simulink model "local_sequencer_harness"  (R2018b)
settings: Solver=FixedStepDiscrete  StartTime=0  StopTime=11  FixedStep=1  RelTol=1e-3
undefined symbols (not defined in the file or in its folder): eof, sigbuilder_block, sldvsubsys, StateFlowModeType
libraries: sldvlib x21, simulink x6, hdlsllib x4
(part 1 of 2)
settings Model: SldvGeneratedHarnessModel=TestUnitModel=local_sequencer|  Creator=hiterd  LastModifiedBy=gauthamsm
settings DataIOCC: SaveFormat=StructureWithTime
settings OptimizationCC: BlockReduction=off  ConditionallyExecuteInputs=off  DefaultParameterBehavior=Inlined  ExpressionFolding=off
settings DebuggingCC: InheritedTsInSrcMsg=none  LibraryContextMissingDiagnostic=none
settings SFSimCC: SimUseLocalCustomCode=off
settings RTWCC: RTWUseLocalCustomCode=off
settings ConfigComp: DVMode=PropertyProving  DVModelCoverageObjectives=MCDC  DVTestSuiteOptimization=CombinedObjectives (Nonlinear Extended)  DVDetectOutOfBounds=on  DVSaveExpectedOutput=on  DVDisplayReport=off

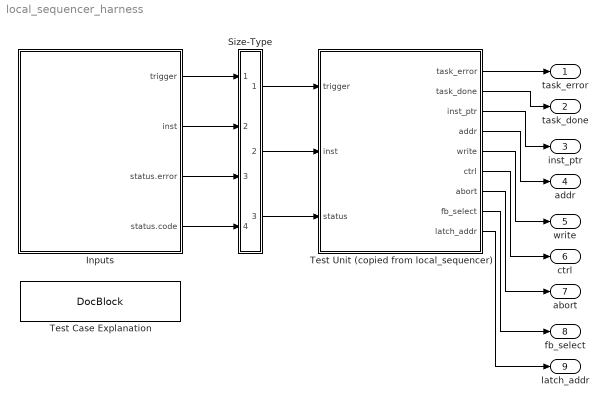
== system local_sequencer_harness ==
  Inputs : Subsystem  Tag=STV Subsys  LoadFcn=sigbuilder_block('load',[50 50 520 400 ]);  StartFcn=sigbuilder_block('start');  StopFcn=sigbuilder_block('stop');  ClipboardFcn=sigbuilder_block('clipboard');  mask(Sigbuilder block){tuvar=[0:10]}
      mask init:
      | if ~strcmp(get_param(bdroot(gcb),'SimulationStatus'),'stopped'),tuvar = sigbuilder_block('maskInit'); end
      settings: CopyFcn=sigbuilder_block('copy');  DeleteFcn=sigbuilder_block('delete');  ModelCloseFcn=sigbuilder_block('modelClose');  PreSaveFcn=sigbuilder_block('preSave');  PauseFcn=sigbuilder_block('pause');  ContinueFcn=sigbuilder_block('continue');  NameChangeFcn=sigbuilder_block('namechange');  OpenFcn=sigbuilder_block('open');  CloseFcn=sigbuilder_block('close');
      mask Display: plot(0, 0, 100, 100,[2, 2, 32, 32, 2], [68, 8, 8, 68, 68],[32, 2], [38, 38], [32, 19, 2],[53, 60, 44], [32, 17, 17, 2],[16, 16, 31, 31]);txt = getActiveGroup(gcbh);text(2, 100, txt,'verticalAlignment', 'top');
  Size-Type : Subsystem
  Test Case Explanation : simulink/Model-Wide Utilities/DocBlock  DocumentType=Text
  Test Unit (copied from local_sequencer) : Subsystem
  task_error : Outport  RequirementInfo={'linktype_rmi_slreq' 'local_sequencer_req.slreqx' '20' 'true' 'ERROR (local_sequencer_req#20)' '' ; 'linktype_rmi_slreq' 'local_sequencer_req.slreqx' '29' 'true' 'Error Signal Service Provided (local_sequencer_req#29)' '' } %GIDa_4b3727b3_eed7_4111_ba54_d506f35d5492  OutDataTypeStr=boolean
  task_done : Outport  RequirementInfo={'linktype_rmi_slreq' 'local_sequencer_req.slreqx' '19' 'true' 'TASK_DONE (local_sequencer_req#19)' '' ; 'linktype_rmi_slreq' 'local_sequencer_req.slreqx' '30' 'true' 'Task Done Service Provided (local_sequencer_req#30)' '' } %GIDa_c01a0f3d_81eb_4c3b_a7a9_b5b96c8ed019  Port=2  OutDataTypeStr=boolean
  inst_ptr : Outport  RequirementInfo={'linktype_rmi_slreq' 'local_sequencer_req.slreqx' '32' 'true' 'Instruction Pointer Service Provided (local_sequencer_req#32)' '' } %GIDa_841fdf6d_6e66_40b6_9879_a3a1e6181a38  Port=3  OutDataTypeStr=task_inst_ptr_type
  addr : Outport  RequirementInfo={'linktype_rmi_slreq' 'local_sequencer_req.slreqx' '31' 'true' 'Task Memory Control Service Provided (local_sequencer_req#31)' '' } %GIDa_8f8748fa_058e_47e8_8fbe_e13b7300a8e2  Port=4  OutMin=[0]  OutDataTypeStr=task_memory_addr_type
  write : Outport  RequirementInfo={'linktype_rmi_slreq' 'local_sequencer_req.slreqx' '17' 'true' 'WRITE (local_sequencer_req#17)' '' ; 'linktype_rmi_slreq' 'local_sequencer_req.slreqx' '31' 'true' 'Task Memory Control Service Provided (local_sequencer_req#31)' '' } %GIDa_4b518ad7_48e7_4af2_afb8_2f880d159183  Port=5  OutDataTypeStr=boolean
  ctrl : Outport  RequirementInfo={'linktype_rmi_slreq' 'local_sequencer_req.slreqx' '15' 'true' 'FETCH (local_sequencer_req#15)' '' ; 'linktype_rmi_slreq' 'local_sequencer_req.slreqx' '16' 'true' 'FB_EXECUTE (local_sequencer_req#16)' '' ; 'linktype_rmi_slreq' 'local_sequencer_req.slreqx' '17' 'true' 'WRITE (local_sequencer_req#17)' '' ; 'linktype_rmi_slreq' 'local_sequencer_req.slreqx' '18' 'true' 'FB_DONE (local_sequencer_req#18)' '' } %GIDa_58b190dd_e50c_4c00_a93b_9cea49031466  Port=6  OutDataTypeStr=boolean
  abort : Outport  RequirementInfo={'linktype_rmi_slreq' 'local_sequencer_req.slreqx' '20' 'true' 'ERROR (local_sequencer_req#20)' '' } %GIDa_8b4e3093_6652_4c1d_818e_447a54a9c3fa  Port=7  OutDataTypeStr=boolean
  fb_select : Outport  RequirementInfo={'linktype_rmi_slreq' 'local_sequencer_req.slreqx' '33' 'true' 'Function Block Selection Service Provided (local_sequencer_req#33)' '' } %GIDa_aec407fa_8f5e_42a9_a8e2_947265fcaaeb  Port=8  OutDataTypeStr=fb_select_type
  latch_addr : Outport  RequirementInfo={} %GIDa_280df430_9f3e_4a55_807b_1e93c9a80428  Port=9  OutMin=[0]  OutDataTypeStr=boolean
  wires:
  Inputs/1(trigger) -> Size-Type/1(In1)
  Size-Type/1(Out1) -> Test Unit (copied from local_sequencer)/1(trigger)
  Inputs/2(inst) -> Size-Type/2(In2)
  Size-Type/2(Out2) -> Test Unit (copied from local_sequencer)/2(inst)
  Inputs/3(status.error) -> Size-Type/3(In5)
  Inputs/4(status.code) -> Size-Type/4(In6)
  Size-Type/3(Out3) -> Test Unit (copied from local_sequencer)/3(status)
  Test Unit (copied from local_sequencer)/1(task_error) -> task_error/1
  Test Unit (copied from local_sequencer)/2(task_done) -> task_done/1
  Test Unit (copied from local_sequencer)/3(inst_ptr) -> inst_ptr/1
  Test Unit (copied from local_sequencer)/4(addr) -> addr/1
  Test Unit (copied from local_sequencer)/5(write) -> write/1
  Test Unit (copied from local_sequencer)/6(ctrl) -> ctrl/1
  Test Unit (copied from local_sequencer)/7(abort) -> abort/1
  Test Unit (copied from local_sequencer)/8(fb_select) -> fb_select/1
  Test Unit (copied from local_sequencer)/9(latch_addr) -> latch_addr/1

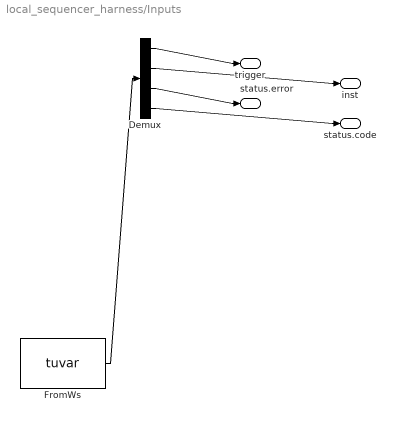
== system local_sequencer_harness/Inputs ==
  Demux : Demux  Tag=STV Demux
  FromWs : FromWorkspace  Tag=STV FromWs  VariableName=tuvar  SampleTime=0
      SigBuilderData=|
      | dataSet(1).timeRange = [0 5]
      | dataSet(1).name = 'Counterexample 1'
      | dataSet(2).timeRange = [0 5]
      | dataSet(2).name = 'Counterexample 2'
      | sbobj.Name = 'Signal Builder'
      | sbobj.Groups(1).Name = 'Counterexample 1'
      | sbobj.Groups(1).Signals(1).Name = 'trigger'
      | sbobj.Groups(1).Signals(1).XData = [0 1 2 3 4 5]
      | sbobj.Groups(1).Signals(1).YData = [1 1 1 1 1 1]
      | sbobj.Groups(1).Signals(2).Name = 'inst'
      | sbobj.Groups(1).Signals(2).XData = [0 1 2 3 4 5]
      | sbobj.Groups(1).Signals(2).YData = [2147483646 2147483646 2147483646 2147483646 2147483646 2147483646]
      | sbobj.Groups(1).Signals(3).Name = 'status.error'
      | sbobj.Groups(1).Signals(3).XData = [0 1 2 3 4 4 5]
      | sbobj.Groups(1).Signals(3).YData = [0 0 0 0 0 1 1]
      | sbobj.Groups(1).Signals(4).Name = 'status.code'
      | sbobj.Groups(1).Signals(4).XData = [0 1 1 2 2 3 3 4 4 5]
      | sbobj.Groups(1).Signals(4).YData = [71303168 71303168 260046849 260046849 524288000 524288000 524288001 524288001 2675965952 2675965952]
      | sbobj.Groups(1).TimeRange = [0 5]
      | sbobj.Groups(2).Name = 'Counterexample 2'
      | sbobj.Groups(2).Signals(1).Name = 'trigger'
      | sbobj.Groups(2).Signals(1).XData = [0 1 2 2 3 3 4 4 5]
      | sbobj.Groups(2).Signals(1).YData = [1 1 1 0 0 1 1 0 0]
      | sbobj.Groups(2).Signals(2).Name = 'inst'
      | sbobj.Groups(2).Signals(2).XData = [0 1 2 3 4 5]
      | sbobj.Groups(2).Signals(2).YData = [2147483646 2147483646 2147483646 2147483646 2147483646 2147483646]
      | sbobj.Groups(2).Signals(3).Name = 'status.error'
      | sbobj.Groups(2).Signals(3).XData = [0 1 2 3 4 4 5]
      | sbobj.Groups(2).Signals(3).YData = [0 0 0 0 0 1 1]
      | sbobj.Groups(2).Signals(4).Name = 'status.code'
      | sbobj.Groups(2).Signals(4).XData = [0 1 1 2 2 3 4 4 5]
      | sbobj.Groups(2).Signals(4).YData = [71303168 71303168 260046848 260046848 524288000 524288000 524288000 2675965953 2675965953]
      | sbobj.Groups(2).TimeRange = [0 5]
  trigger : Outport  Tag=STV Outport
  inst : Outport  Tag=STV Outport  Port=2
  status.error : Outport  Tag=STV Outport  Port=3
  status.code : Outport  Tag=STV Outport  Port=4
  wires:
  FromWs/1 -> Demux/1
  Demux/1 -> trigger/1
  Demux/2 -> inst/1
  Demux/3 -> status.error/1
  Demux/4 -> status.code/1

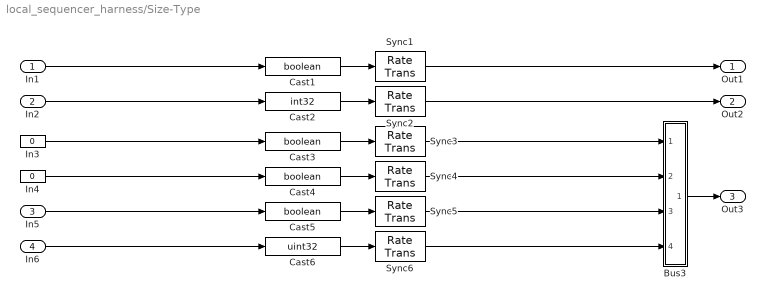
== system local_sequencer_harness/Size-Type ==
  In1 : Inport
  In2 : Inport  Port=2
  In5 : Inport  Port=3
  In6 : Inport  Port=4
  Bus3 : Subsystem
  Cast{1,3..5} (4 alike) : DataTypeConversion  OutDataTypeStr=boolean  RndMeth=Nearest  SaturateOnIntegerOverflow=on
  Cast2 : DataTypeConversion  OutDataTypeStr=int32  RndMeth=Nearest  SaturateOnIntegerOverflow=on
  Cast6 : DataTypeConversion  OutDataTypeStr=uint32  RndMeth=Nearest  SaturateOnIntegerOverflow=on
  In3 : Constant  Value=0  OutDataTypeStr=double
  In4 : Constant  Value=0  OutDataTypeStr=double
  Sync{1..6} (6 alike) : RateTransition  OutPortSampleTime=[1,0]
  Out1 : Outport
  Out2 : Outport  Port=2
  Out3 : Outport  Port=3
  wires:
  In1/1 -> Cast1/1
  Cast1/1 -> Sync1/1
  Sync1/1 -> Out1/1
  In2/1 -> Cast2/1
  Cast2/1 -> Sync2/1
  Sync2/1 -> Out2/1
  In3/1 -> Cast3/1
  Cast3/1 -> Sync3/1
  In4/1 -> Cast4/1
  Cast4/1 -> Sync4/1
  In5/1 -> Cast5/1
  Cast5/1 -> Sync5/1
  In6/1 -> Cast6/1
  Cast6/1 -> Sync6/1
  Sync3/1 -> Bus3/1(status(1).done)
  Sync4/1 -> Bus3/2(status(1).busy)
  Sync5/1 -> Bus3/3(status(1).error)
  Sync6/1 -> Bus3/4(status(1).code)
  Bus3/1(Out) -> Out3/1

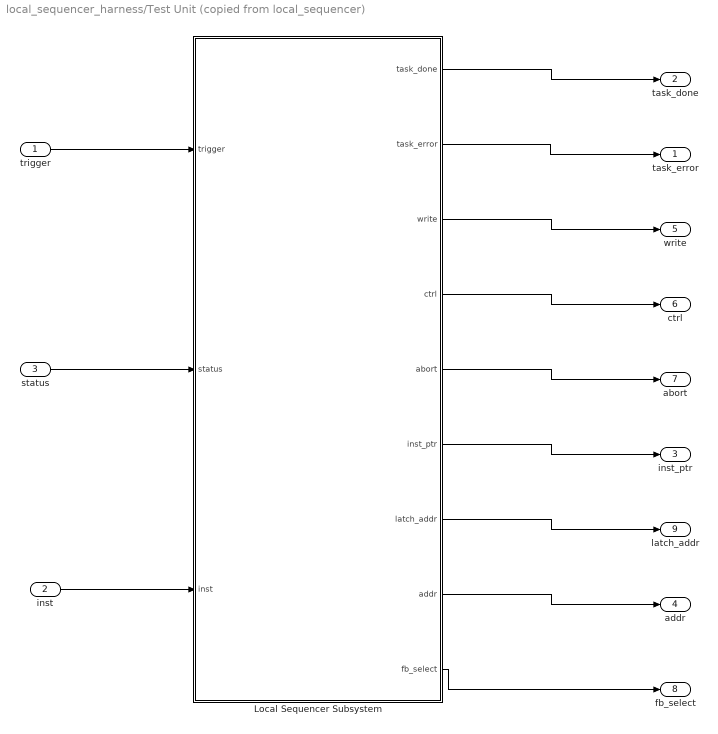
== system local_sequencer_harness/Test Unit (copied from local_sequencer) ==
  trigger : Inport  RequirementInfo={'linktype_rmi_slreq' 'local_sequencer_req.slreqx' '1' 'true' 'Trigger Service Received (local_sequencer_req#1)' '' } %GIDa_4d9765d8_c1f7_44d1_847e_63d15330923d  OutDataTypeStr=boolean  SampleTime=1
  inst : Inport  RequirementInfo={'linktype_rmi_slreq' 'local_sequencer_req.slreqx' '2' 'true' 'Instruction Service Received (local_sequencer_req#2)' '' } %GIDa_6e08ed8d_7128_4ad3_9be2_20afc87b0780  Port=2  OutDataTypeStr=task_inst_data_type  SampleTime=1
  status : Inport  RequirementInfo={'linktype_rmi_slreq' 'local_sequencer_req.slreqx' '3' 'true' 'Function Block Status Service Received (local_sequencer_req#3)' '' } %GIDa_a844bf10_1c01_4e71_b367_abd6e060c4a4  Port=3  OutDataTypeStr=Bus: fb_status  SampleTime=1
  Local Sequencer Subsystem : Subsystem  RequirementInfo={} %GIDa_691ea0b4_f849_451b_b844_cf268bee6922
  task_error : Outport  RequirementInfo={'linktype_rmi_slreq' 'local_sequencer_req.slreqx' '20' 'true' 'ERROR (local_sequencer_req#20)' '' ; 'linktype_rmi_slreq' 'local_sequencer_req.slreqx' '29' 'true' 'Error Signal Service Provided (local_sequencer_req#29)' '' } %GIDa_e9ce8bc7_3977_4377_8523_e6d870486e24  OutDataTypeStr=boolean
  task_done : Outport  RequirementInfo={'linktype_rmi_slreq' 'local_sequencer_req.slreqx' '19' 'true' 'TASK_DONE (local_sequencer_req#19)' '' ; 'linktype_rmi_slreq' 'local_sequencer_req.slreqx' '30' 'true' 'Task Done Service Provided (local_sequencer_req#30)' '' } %GIDa_4f63a98d_be6f_4c69_865c_747d34c7a994  Port=2  OutDataTypeStr=boolean
  inst_ptr : Outport  RequirementInfo={'linktype_rmi_slreq' 'local_sequencer_req.slreqx' '32' 'true' 'Instruction Pointer Service Provided (local_sequencer_req#32)' '' } %GIDa_ae4a976f_0dc8_4a2d_b976_c9d40035a665  Port=3  OutDataTypeStr=task_inst_ptr_type
  addr : Outport  RequirementInfo={'linktype_rmi_slreq' 'local_sequencer_req.slreqx' '31' 'true' 'Task Memory Control Service Provided (local_sequencer_req#31)' '' } %GIDa_c8e29bee_29f9_4d2c_a739_7a936b29a70c  Port=4  OutMin=[0]  OutDataTypeStr=task_memory_addr_type
  write : Outport  RequirementInfo={'linktype_rmi_slreq' 'local_sequencer_req.slreqx' '17' 'true' 'WRITE (local_sequencer_req#17)' '' ; 'linktype_rmi_slreq' 'local_sequencer_req.slreqx' '31' 'true' 'Task Memory Control Service Provided (local_sequencer_req#31)' '' } %GIDa_a08e580f_e59d_4d36_808e_415d3b412f66  Port=5  OutDataTypeStr=boolean
  ctrl : Outport  RequirementInfo={'linktype_rmi_slreq' 'local_sequencer_req.slreqx' '15' 'true' 'FETCH (local_sequencer_req#15)' '' ; 'linktype_rmi_slreq' 'local_sequencer_req.slreqx' '16' 'true' 'FB_EXECUTE (local_sequencer_req#16)' '' ; 'linktype_rmi_slreq' 'local_sequencer_req.slreqx' '17' 'true' 'WRITE (local_sequencer_req#17)' '' ; 'linktype_rmi_slreq' 'local_sequencer_req.slreqx' '18' 'true' 'FB_DONE (local_sequencer_req#18)' '' } %GIDa_798b687a_16a8_42b6_9002_483e38f3c64e  Port=6  OutDataTypeStr=boolean
  abort : Outport  RequirementInfo={'linktype_rmi_slreq' 'local_sequencer_req.slreqx' '20' 'true' 'ERROR (local_sequencer_req#20)' '' } %GIDa_0f3d61c3_2d7b_4dce_ac88_a1459569f952  Port=7  OutDataTypeStr=boolean
  fb_select : Outport  RequirementInfo={'linktype_rmi_slreq' 'local_sequencer_req.slreqx' '33' 'true' 'Function Block Selection Service Provided (local_sequencer_req#33)' '' } %GIDa_2bafbd9a_e614_424c_a6eb_704ceba625c2  Port=8  OutDataTypeStr=fb_select_type
  latch_addr : Outport  RequirementInfo={} %GIDa_f6d0df7c_bed9_4f3c_a302_54711bc6950e  Port=9  OutMin=[0]  OutDataTypeStr=boolean
  wires:
  trigger/1 -> Local Sequencer Subsystem/1(trigger)
  status/1 -> Local Sequencer Subsystem/2(status)
  inst/1 -> Local Sequencer Subsystem/3(inst)
  Local Sequencer Subsystem/1(task_done) -> task_done/1
  Local Sequencer Subsystem/2(task_error) -> task_error/1
  Local Sequencer Subsystem/3(write) -> write/1
  Local Sequencer Subsystem/4(ctrl) -> ctrl/1
  Local Sequencer Subsystem/5(abort) -> abort/1
  Local Sequencer Subsystem/6(inst_ptr) -> inst_ptr/1
  Local Sequencer Subsystem/7(latch_addr) -> latch_addr/1
  Local Sequencer Subsystem/8(addr) -> addr/1
  Local Sequencer Subsystem/9(fb_select) -> fb_select/1

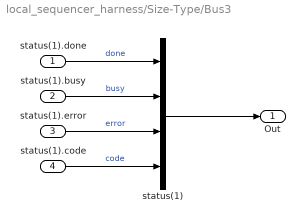
== system local_sequencer_harness/Size-Type/Bus3 ==
  status(1).done : Inport
  status(1).busy : Inport  Port=2
  status(1).error : Inport  Port=3
  status(1).code : Inport  Port=4
  status(1) : BusCreator  Inputs=4  OutDataTypeStr=Bus: fb_status
  Out : Outport
  wires:
  status(1).done/1 -> status(1)/1  "done"
  status(1).busy/1 -> status(1)/2  "busy"
  status(1).error/1 -> status(1)/3  "error"
  status(1).code/1 -> status(1)/4  "code"
  status(1)/1 -> Out/1

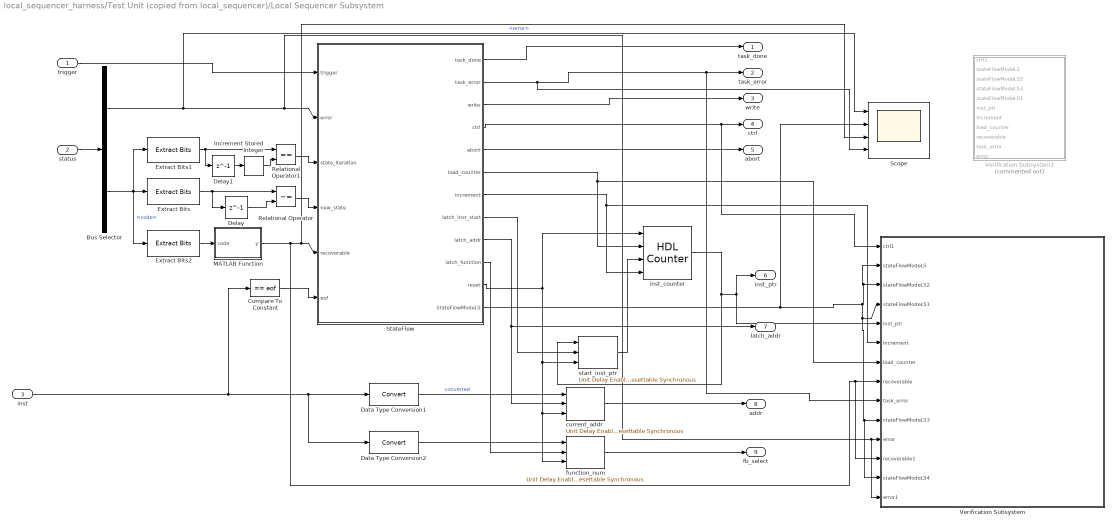
== system local_sequencer_harness/Test Unit (copied from local_sequencer)/Local Sequencer Subsystem ==
  trigger : Inport  RequirementInfo={} %GIDa_1e8ca34a_c9d3_45ae_b0e7_559df57917bf
  status : Inport  RequirementInfo={} %GIDa_1a7e6c0b_3888_45e7_9699_00d25f52f0df  Port=2
  inst : Inport  RequirementInfo={} %GIDa_cf2bd6e1_6b2b_450c_945a_cc71645fdc78  Port=3
  Bus Selector : BusSelector  RequirementInfo={} %GIDa_a162605f_6826_4012_8456_0f670d372e3e  OutputSignals=error,code
  Compare To Constant : simulink/Logic and Bit Operations/Compare To Constant  RequirementInfo={'linktype_rmi_slreq' 'local_sequencer_req.slreqx' '7' 'true' 'End of File Determination (local_sequencer_req#7)' '' } %GIDa_1bfea16f_c62a_4475_9710_996025bad8c0  relop===  const=eof  OutDataTypeStr=boolean
  Data Type Conversion1 : DataTypeConversion  RequirementInfo={'linktype_rmi_slreq' 'local_sequencer_req.slreqx' '34' 'true' 'Conversion of Data Input (local_sequencer_req#34)' '' } %GIDa_bcea22fb_1305_4e6d_9be5_7c5894791e9c
  Data Type Conversion2 : DataTypeConversion  RequirementInfo={'linktype_rmi_slreq' 'local_sequencer_req.slreqx' '34' 'true' 'Conversion of Data Input (local_sequencer_req#34)' '' } %GIDa_b03bb29e_727f_4560_91c2_987e1544289f
  Delay : Delay  RequirementInfo={'linktype_rmi_slreq' 'local_sequencer_req.slreqx' '5' 'true' 'Super State Change Detection (local_sequencer_req#5)' '' } %GIDa_826e27ed_e26c_448f_bb39_3b3ecfac7830  DelayLength=1
  Delay1 : Delay  RequirementInfo={'linktype_rmi_slreq' 'local_sequencer_req.slreqx' '4' 'true' 'Super State Iteration Detection (local_sequencer_req#4)' '' } %GIDa_9af56f70_0ad9_4e15_b1d3_d222492c0231  DelayLength=1
  Extract Bits : simulink/Logic and Bit Operations/Extract Bits  RequirementInfo={'linktype_rmi_slreq' 'local_sequencer_req.slreqx' '5' 'true' 'Super State Change Detection (local_sequencer_req#5)' '' } %GIDa_ed216d48_4236_4a6e_94ae_32688075c1c1  bitsToExtract=Range starting with most significant bit  numBits=4  bitIdxRange=[0 7]  outScalingMode=Treat bit field as an integer
      settings: SourceProductName=Simulink
  Extract Bits1 : simulink/Logic and Bit Operations/Extract Bits  RequirementInfo={'linktype_rmi_slreq' 'local_sequencer_req.slreqx' '4' 'true' 'Super State Iteration Detection (local_sequencer_req#4)' '' } %GIDa_f8a72584_cc2f_4dda_9538_a363ad475483  bitsToExtract=Range of bits  numBits=4  bitIdxRange=[22 27]  outScalingMode=Treat bit field as an integer
      settings: SourceProductName=Simulink
  Extract Bits2 : simulink/Logic and Bit Operations/Extract Bits  RequirementInfo={'linktype_rmi_slreq' 'local_sequencer_req.slreqx' '6' 'true' 'Error Recovery Determination (local_sequencer_req#6)' '' } %GIDa_6508cd16_8925_49b2_89d0_f2044608e5fd  bitsToExtract=Range ending with least significant bit  numBits=22  bitIdxRange=[22 27]  outScalingMode=Treat bit field as an integer
      settings: SourceProductName=Simulink
  Increment Stored Integer : simulink/Additional Math & Discrete/Additional Math: Increment - Decrement/Increment Stored Integer  RequirementInfo={'linktype_rmi_slreq' 'local_sequencer_req.slreqx' '4' 'true' 'Super State Iteration Detection (local_sequencer_req#4)' '' } %GIDa_eff492e6_55b4_4f8f_bf38_25fea0c3ba44
      settings: SourceProductName=Simulink
  MATLAB Function : MATLAB Function  RequirementInfo={'linktype_rmi_slreq' 'local_sequencer_req.slreqx' '6' 'true' 'Error Recovery Determination (local_sequencer_req#6)' '' } %GIDa_0e0ae0c6_7f44_44d8_8ce2_7f424de04522  TreatAsAtomicUnit=on
  Relational Operator : RelationalOperator  RequirementInfo={'linktype_rmi_slreq' 'local_sequencer_req.slreqx' '5' 'true' 'Super State Change Detection (local_sequencer_req#5)' '' } %GIDa_c7a5acef_9ee6_48bf_acb3_5cd08911dcb3  Operator=~=  OutDataTypeStr=boolean  RndMeth=Nearest
  Relational Operator1 : RelationalOperator  RequirementInfo={'linktype_rmi_slreq' 'local_sequencer_req.slreqx' '4' 'true' 'Super State Iteration Detection (local_sequencer_req#4)' '' } %GIDa_e00291a7_d6c4_4999_8243_fd86dde3d581  Operator===  OutDataTypeStr=boolean  RndMeth=Nearest
  Scope : Scope  NumInputPorts=4
      settings: RequirementInfo={} %GIDa_a27e6c01_8b88_4284_ab1b_80a338979146
  StateFlow : Stateflow chart  RequirementInfo={'linktype_rmi_slreq' 'local_sequencer_req.slreqx' '12' 'true' 'Controller Super States (local_sequencer_req#12)' '' } %GIDa_cc643d51_32d6_41cb_beee_853cbc937ec5  TreatAsAtomicUnit=on
  Verification Subsystem : Subsystem  Tag=VerificationSubsystem  RequirementInfo={} %GIDa_b9231509_133e_4ec9_afa8_12fadf576824  DisableCoverage=on  LoadFcn=sldvsubsys('check')  TreatAsAtomicUnit=on  SimViewingDevice=on  mask(VerificationSubsystem){}
      mask init:
      | sldvsubsys('maskInit');
      settings: CopyFcn=sldvsubsys('copy');  OpenFcn=open_system(gcb,'force');
      settings: PreSaveFcn=|
      | set_param(gcb,'SimViewingDevice','on');
      | sldvsubsys('check');
      mask Help: helpview(fullfile(docroot,'toolbox','sldv','sldv.map'),'verificationsubsystem')
      mask Display: image(imread('sldvicon_versubsys.png','BackGroundColor',[1 1 1]),'center');
  Verification Subsystem1 : Subsystem  Tag=VerificationSubsystem  RequirementInfo={} %GIDa_b5211482_203e_477a_a04f_44f6097f9954  Commented=on  DisableCoverage=on  LoadFcn=sldvsubsys('check')  TreatAsAtomicUnit=on  SimViewingDevice=on  mask(VerificationSubsystem){}
      mask init:
      | sldvsubsys('maskInit');
      settings: CopyFcn=sldvsubsys('copy');  OpenFcn=open_system(gcb,'force');
      settings: PreSaveFcn=|
      | set_param(gcb,'SimViewingDevice','on');
      | sldvsubsys('check');
      mask Help: helpview(fullfile(docroot,'toolbox','sldv','sldv.map'),'verificationsubsystem')
      mask Display: image(imread('sldvicon_versubsys.png','BackGroundColor',[1 1 1]),'center');
  current_addr : hdlsllib/Discrete/Unit Delay Enabled Resettable Synchronous  RequirementInfo={'linktype_rmi_slreq' 'local_sequencer_req.slreqx' '11' 'true' 'Current Address Register (local_sequencer_req#11)' '' } %GIDa_b8f7f4f3_37ca_4546_8bdc_9675d816c663  InitialCondition=0  SampleTime=-1
      settings: SourceProductName=HDL Coder  SourceProductBaseCode=HD
  function_num : hdlsllib/Discrete/Unit Delay Enabled Resettable Synchronous  RequirementInfo={'linktype_rmi_slreq' 'local_sequencer_req.slreqx' '8' 'true' 'Function Number Register (local_sequencer_req#8)' '' } %GIDa_658e3425_55a5_4c8c_8b70_ff26cff3d567  InitialCondition=0  SampleTime=-1
      settings: SourceProductName=HDL Coder  SourceProductBaseCode=HD
  inst_counter : hdlsllib/Sources/HDL Counter  RequirementInfo={'linktype_rmi_slreq' 'local_sequencer_req.slreqx' '10' 'true' 'Instruction Counter (local_sequencer_req#10)' '' } %GIDa_4f8fbdf8_b7e8_445f_8c6c_70eaab5f3fef  CountType=Free running  CountInit=0  CountStep=1  CountMax=25  CountFromType=Initial value  CountFrom=0  CountResetPort=on  CountLoadPort=on  CountEnbPort=on  CountDirPort=off  CountDataType=Unsigned  CountWordLen=32  CountFracLen=0  CountSampTime=1
      settings: SourceProductBaseCode=HD
  start_inst_ptr : hdlsllib/Discrete/Unit Delay Enabled Resettable Synchronous  RequirementInfo={'linktype_rmi_slreq' 'local_sequencer_req.slreqx' '9' 'true' 'Start Instruction Pointer Register (local_sequencer_req#9)' '' } %GIDa_059fbd8a_63b8_486f_a2ee_beef95e9e77a  InitialCondition=0  SampleTime=-1
      settings: SourceProductName=HDL Coder  SourceProductBaseCode=HD
  task_done : Outport  RequirementInfo={} %GIDa_742b0145_7b38_4077_85b0_9b3c6bbcc75a
  task_error : Outport  RequirementInfo={} %GIDa_20ca7631_3271_4d84_8143_ec18b5855ad9  Port=2
  write : Outport  RequirementInfo={} %GIDa_15c2c95f_69ed_4817_8697_d9e8efe15443  Port=3
  ctrl : Outport  RequirementInfo={} %GIDa_ab925feb_6031_4560_b0bf_8fccdac808d1  Port=4
  abort : Outport  RequirementInfo={} %GIDa_af91d9c3_b667_48b7_844a_d06301abb7fe  Port=5
  inst_ptr : Outport  RequirementInfo={} %GIDa_92246ee0_b390_431d_84f7_855d2625f298  Port=6
  latch_addr : Outport  RequirementInfo={} %GIDa_c018af9e_064e_4093_9f4e_4119ccab6bc1  Port=7
  addr : Outport  RequirementInfo={} %GIDa_55309190_ab2c_44a1_af5f_111a38240509  Port=8
  fb_select : Outport  RequirementInfo={} %GIDa_d0ad82d1_5299_4359_b05c_642c3938d8a5  Port=9
  wires:
  StateFlow/12(StateFlowModeLS) -> Verification Subsystem/2(stateFlowModeLS), Verification Subsystem/3(stateFlowModeLS2), Verification Subsystem/4(stateFlowModeLS1), Verification Subsystem/10(stateFlowModeLS3), Verification Subsystem/13(stateFlowModeLS4), Scope/2
  StateFlow/3(write) -> write/1
  current_addr/1 -> addr/1
  StateFlow/4(ctrl) -> ctrl/1, Verification Subsystem/1(ctrl1)
  StateFlow/1(task_done) -> task_done/1
  trigger/1 -> StateFlow/1(trigger)
  Extract Bits/1 -> Delay/1, Relational Operator/1
  MATLAB Function/1(y) -> StateFlow/5(recoverable), Scope/3, Verification Subsystem/8(recoverable), Verification Subsystem/12(recoverable1)
  StateFlow/10(latch_function) -> function_num/2
  Data Type Conversion2/1 -> function_num/1
  Relational Operator1/1 -> StateFlow/3(state_iteration)
  Delay/1 -> Relational Operator/2
  StateFlow/2(task_error) -> task_error/1, Verification Subsystem/9(task_error), Scope/4
  function_num/1 -> fb_select/1
  inst/1 -> Compare To Constant/1, Data Type Conversion2/1, Data Type Conversion1/1
  Compare To Constant/1 -> StateFlow/6(eof)
  Relational Operator/1 -> StateFlow/4(new_state)
  Bus Selector/1 -> StateFlow/2(error), Verification Subsystem/11(error), Verification Subsystem/14(error1), Scope/1  "<error>"
  inst_counter/1 -> start_inst_ptr/1, inst_ptr/1, Verification Subsystem/5(inst_ptr)
  Increment Stored Integer/1 -> Relational Operator1/2
  Delay1/1 -> Increment Stored Integer/1
  StateFlow/5(abort) -> abort/1
  Extract Bits1/1 -> Relational Operator1/1, Delay1/1
  Extract Bits2/1 -> MATLAB Function/1(code)
  Bus Selector/2 -> Extract Bits/1, Extract Bits1/1, Extract Bits2/1  "<code>"
  StateFlow/6(load_counter) -> inst_counter/2, Verification Subsystem/7(load_counter)
  StateFlow/11(reset) -> inst_counter/1, start_inst_ptr/3, current_addr/3, function_num/3
  start_inst_ptr/1 -> inst_counter/3
  Data Type Conversion1/1 -> current_addr/1  "converted"
  status/1 -> Bus Selector/1
  StateFlow/7(increment) -> inst_counter/4, Verification Subsystem/6(increment)
  StateFlow/8(latch_inst_start) -> start_inst_ptr/2
  StateFlow/9(latch_addr) -> current_addr/2, latch_addr/1

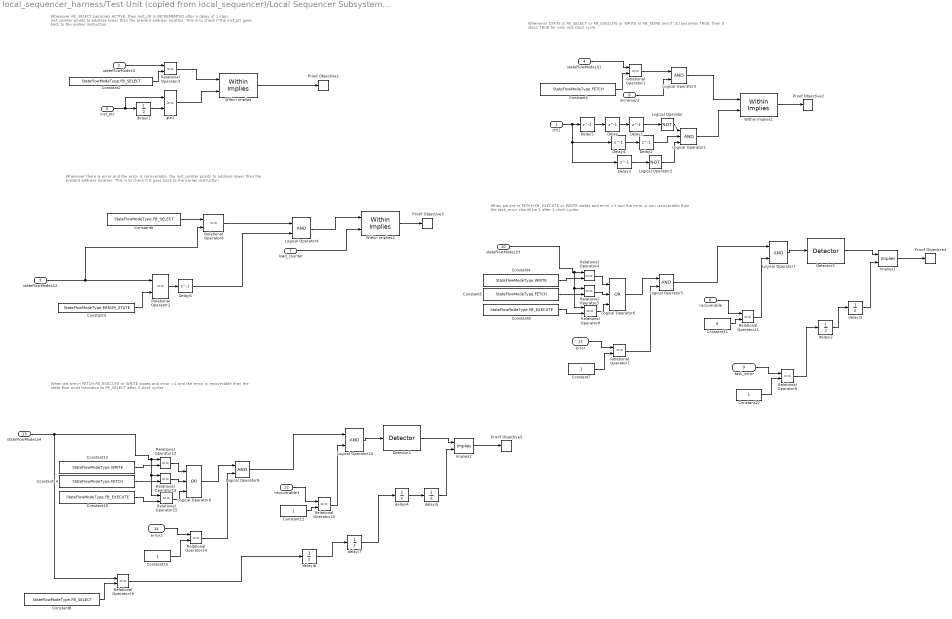
== system local_sequencer_harness/Test Unit (copied from local_sequencer)/Local Sequencer Subsystem/Verification Subsystem ==
  note: When we are in FETCH,FB_EXECUTE or WRITE states and error =1 and the error is
      | recoverable then the state flow must transition to FB_SELECT after 3 clock cycles
  note: When we are in FETCH,FB_EXECUTE or WRITE states and error =1 and the error is non
      | recoverable then the task_error should be 1 after 2 clock cycles
  note: Whenever there is error and the error is recoverable, the inst_pointer points to address lower than the present address location. This is to check if it goes back to the earlier instruction
  note: Whenever STATE is FB_SELECT or FB_EXECUTE or WRITE or FB_DONE and if ctrl becomes TRUE, then it stays TRUE for only one clock cycle.
  note: Whenever FB_SELECT becomes ACTIVE, then inst_ptr is INCREMENTED after a delay of 1 step. inst_pointer points to address lower than the present address location. This is to check if the inst_ptr goes back to the earlier instruction
  ctrl1 : Inport  RequirementInfo={} %GIDa_6b645b52_a750_41af_9a8f_c377cd2cb97e
  stateFlowModeLS : Inport  RequirementInfo={} %GIDa_a4712168_761f_42ae_85b8_8ff9b981d0c1  Port=2  OutDataTypeStr=Enum: StateFlowModeType
  stateFlowModeLS2 : Inport  RequirementInfo={} %GIDa_a7c47b6a_432f_4217_84f3_98ed5b16bf25  Port=3  OutDataTypeStr=Enum: StateFlowModeType
  stateFlowModeLS1 : Inport  RequirementInfo={} %GIDa_5f3d4289_f256_4d9b_bbfa_4cb2e9ba7701  Port=4  OutDataTypeStr=Enum: StateFlowModeType
  inst_ptr : Inport  RequirementInfo={} %GIDa_c73084db_e622_4a82_be5c_67d8c46f613f  Port=5
  increment : Inport  RequirementInfo={} %GIDa_34715739_1965_4b88_a576_10e1b9c7bcf1  Port=6
  load_counter : Inport  RequirementInfo={} %GIDa_5349dcb2_c6d2_4b2e_b931_b803d0eafd2b  Port=7
  recoverable : Inport  RequirementInfo={} %GIDa_52514d1c_d4b4_450c_86d9_102baf416947  Port=8
  task_error : Inport  RequirementInfo={} %GIDa_964329ab_c3cb_483d_bd3e_3f8fce772734  Port=9
  stateFlowModeLS3 : Inport  RequirementInfo={} %GIDa_9f2c847c_a6f0_4dc8_bb70_fd807a5031c3  Port=10  OutDataTypeStr=Enum: StateFlowModeType
  error : Inport  RequirementInfo={} %GIDa_04b1a319_44c2_495c_839e_7cc0812e627f  Port=11
  recoverable1 : Inport  RequirementInfo={} %GIDa_8b8bdee0_7233_4c53_b78f_8a52cb74d75c  Port=12
  stateFlowModeLS4 : Inport  RequirementInfo={} %GIDa_8e458654_ea3c_4d4d_a88e_c6df996ebab2  Port=13  OutDataTypeStr=Enum: StateFlowModeType
  error1 : Inport  RequirementInfo={} %GIDa_44510cdf_839a_486d_8342_15fd6b9a6cb1  Port=14
  Constant1 : Constant  RequirementInfo={} %GIDa_6342d419_8342_43a0_919e_6a27c2e3eafb  Value=StateFlowModeType.FETCH
  Constant10 : Constant  RequirementInfo={} %GIDa_71987e0a_f819_4bc1_ae0f_86cb959ba58c
  Constant11 : Constant  RequirementInfo={} %GIDa_53afce07_30fd_4890_a83f_b84bd58684b9  Value=0
  Constant12 : Constant  RequirementInfo={} %GIDa_03f01666_acfc_4a3b_baa9_c0a59d7d126e
  Constant13 : Constant  RequirementInfo={} %GIDa_e2c573b3_bc29_4365_a3fd_1284c1938177  Value=StateFlowModeType.WRITE
  Constant14 : Constant  RequirementInfo={} %GIDa_779f599a_1458_40c4_9c18_37dc7796f943  Value=StateFlowModeType.FETCH
  Constant15 : Constant  RequirementInfo={} %GIDa_dcb54f72_e8f5_4e18_8b8c_1ce10482da3a
  Constant16 : Constant  RequirementInfo={} %GIDa_e11c02e6_61a8_4c9a_98bf_78bf0f833513  Value=StateFlowModeType.FB_EXECUTE
  Constant2 : Constant  RequirementInfo={} %GIDa_d77b991c_77a2_43c8_ba8b_1d5970f428ac  Value=StateFlowModeType.FB_SELECT
  Constant3 : Constant  RequirementInfo={} %GIDa_d4a9d497_af6c_46f0_916a_43b417355251  Value=StateFlowModeType.ERROR_STATE
  Constant4 : Constant  RequirementInfo={} %GIDa_1e8e59d8_61df_4eca_8fc5_fa09a17b912f  Value=StateFlowModeType.WRITE
  Constant5 : Constant  RequirementInfo={} %GIDa_aae79a7f_f71c_4685_826d_81802dfd129c  Value=StateFlowModeType.FETCH
  Constant6 : Constant  RequirementInfo={} %GIDa_0c059a54_d970_4c46_8833_35b3baf3127a  Value=StateFlowModeType.FB_SELECT
  Constant7 : Constant  RequirementInfo={} %GIDa_a0429521_ac1f_4e13_ac01_d69038e9b625
  Constant8 : Constant  RequirementInfo={} %GIDa_ccd36f88_2729_4a8b_ae6c_3d5c45613874  Value=StateFlowModeType.FB_SELECT
  Constant9 : Constant  RequirementInfo={} %GIDa_e96794ef_4892_4db9_b2c5_07e7e6a3d411  Value=StateFlowModeType.FB_EXECUTE
  Delay : Delay  RequirementInfo={} %GIDa_81740ed4_2784_46f4_85c1_6dbb980f36f6  DelayLength=1  InitialCondition=0
  Delay1 : Delay  RequirementInfo={} %GIDa_dffa4db5_9115_4a6c_bc24_8c31b2b0ae2a  DelayLength=1  InitialCondition=0
  Delay2 : Delay  RequirementInfo={} %GIDa_2b4b34b7_28e3_4da6_9c5c_4161cd76c929  DelayLength=1  InitialCondition=0
  Delay3 : Delay  RequirementInfo={} %GIDa_270c8dcf_c5d6_488c_ab8a_01f21eeed551  DelayLength=1  InitialCondition=0
  Delay4 : Delay  RequirementInfo={} %GIDa_dbf84748_c074_4f31_a9ee_19102cc2667d  DelayLength=1  InitialCondition=0
  Delay5 : Delay  RequirementInfo={} %GIDa_a0fa6fc2_72eb_4e0f_a7af_2b7f78e5a878  DelayLength=1  InitialCondition=0
  Delay6 : Delay  RequirementInfo={} %GIDa_5fa518e1_4830_403b_ae9c_a2474cbcca20  DelayLength=1  InitialCondition=0
  Detector1 : sldvlib/Temporal Operators/Detector  RequirementInfo={} %GIDa_c502c215_ee6c_43d8_964a_396c216b10d4  reset=off  typ=Synchronized  in_hold=1  delay=0  out_hold=5
      settings: SourceProductName=Simulink Design Verifier  SourceProductBaseCode=DV
  Detector3 : sldvlib/Temporal Operators/Detector  RequirementInfo={} %GIDa_429b4896_adea_437f_bd01_5c74a7223186  reset=off  typ=Synchronized  in_hold=1  delay=0  out_hold=5
      settings: SourceProductName=Simulink Design Verifier  SourceProductBaseCode=DV
  Implies1 : sldvlib/Verification Utilities/Implies  RequirementInfo={} %GIDa_bcc7acba_1732_4f58_86db_9c51ed75f38e
      settings: SourceProductName=Simulink Design Verifier  SourceProductBaseCode=DV
  Implies2 : sldvlib/Verification Utilities/Implies  RequirementInfo={} %GIDa_3da248e8_263d_4261_900c_bf2069b027ae
      settings: SourceProductName=Simulink Design Verifier  SourceProductBaseCode=DV
  Logical Operator : Logic  RequirementInfo={} %GIDa_c6ed2fd7_7032_49f1_a73b_59b232d92cfa  Operator=NOT  AllPortsSameDT=off  OutDataTypeStr=boolean
  Logical Operator1 : Logic  RequirementInfo={} %GIDa_11b62c84_4c5b_4fff_b035_221ee7236042  Inputs=3  AllPortsSameDT=off  OutDataTypeStr=boolean
  Logical Operator10 : Logic  RequirementInfo={} %GIDa_82e77056_138f_472c_b35d_04f729bcb552  AllPortsSameDT=off  OutDataTypeStr=boolean
  Logical Operator2 : Logic  RequirementInfo={} %GIDa_bee70a3f_34a4_42dd_b4fe_8c7d25cafb6e  Operator=NOT  AllPortsSameDT=off  OutDataTypeStr=boolean
  Logical Operator3 : Logic  RequirementInfo={} %GIDa_c04f8a76_e51d_4572_9eaa_1319f3d004e1  AllPortsSameDT=off  OutDataTypeStr=boolean
  Logical Operator4 : Logic  RequirementInfo={} %GIDa_ab3c7ee4_4ec3_48d2_9d3e_592908a914fb  AllPortsSameDT=off  OutDataTypeStr=boolean
  Logical Operator5 : Logic  RequirementInfo={} %GIDa_ca91440f_2aa8_4db9_ae7e_a8e1b3d85a5f  AllPortsSameDT=off  OutDataTypeStr=boolean
  Logical Operator6 : Logic  RequirementInfo={} %GIDa_4e9b8a00_7f15_48ae_9c5a_83dd16d3023f  Operator=OR  Inputs=3  AllPortsSameDT=off  OutDataTypeStr=boolean
  Logical Operator7 : Logic  RequirementInfo={} %GIDa_d4822b1c_c277_4986_8ef2_0ba86d669a9a  AllPortsSameDT=off  OutDataTypeStr=boolean
  Logical Operator8 : Logic  RequirementInfo={} %GIDa_59985dd0_0c9a_462a_968b_9254ac594ae7  AllPortsSameDT=off  OutDataTypeStr=boolean
  Logical Operator9 : Logic  RequirementInfo={} %GIDa_0dbbede8_9d83_420c_8489_53d8464b74de  Operator=OR  Inputs=3  AllPortsSameDT=off  OutDataTypeStr=boolean
  Proof Objective1 : sldvlib/Objectives and Constraints/Proof Objective  RequirementInfo={} %GIDa_5a0a3da4_26cd_474e_a9c3_b72501387497  enabled=on  customAVTBlockType=Proof Objective  intervals=true  dispValues=on  outEnabled=off  enableStopSim=off
      settings: AttributesFormatString=%<intervals>  SourceProductName=Simulink Design Verifier  SourceProductBaseCode=DV
  Proof Objective2 : sldvlib/Objectives and Constraints/Proof Objective  RequirementInfo={} %GIDa_d2226da2_0640_43ab_b532_66cb5d7be1b4  enabled=on  customAVTBlockType=Proof Objective  intervals=true  dispValues=on  outEnabled=off  enableStopSim=off
      settings: AttributesFormatString=%<intervals>  SourceProductName=Simulink Design Verifier  SourceProductBaseCode=DV
  Proof Objective3 : sldvlib/Objectives and Constraints/Proof Objective  RequirementInfo={} %GIDa_01fe3c8b_43be_4698_aaaa_97b4f297ef17  enabled=on  customAVTBlockType=Proof Objective  intervals=true  dispValues=on  outEnabled=off  enableStopSim=off
      settings: AttributesFormatString=%<intervals>  SourceProductName=Simulink Design Verifier  SourceProductBaseCode=DV
  Proof Objective4 : sldvlib/Objectives and Constraints/Proof Objective  RequirementInfo={} %GIDa_9469e876_a232_4cd3_b85f_012dd7833a7e  enabled=on  customAVTBlockType=Proof Objective  intervals=true  dispValues=on  outEnabled=off  enableStopSim=off
      settings: AttributesFormatString=%<intervals>  SourceProductName=Simulink Design Verifier  SourceProductBaseCode=DV
  Proof Objective5 : sldvlib/Objectives and Constraints/Proof Objective  RequirementInfo={} %GIDa_7d698c32_5674_4f5c_b6ac_03b8d8626e4d  enabled=on  customAVTBlockType=Proof Objective  intervals=true  dispValues=on  outEnabled=off  enableStopSim=off
      settings: AttributesFormatString=%<intervals>  SourceProductName=Simulink Design Verifier  SourceProductBaseCode=DV
  Relational Operator1 : RelationalOperator  RequirementInfo={} %GIDa_05c76a94_f4f3_4cb4_bfc3_a5737cdb0e00  Operator===  OutDataTypeStr=boolean  RndMeth=Nearest
  Relational Operator10 : RelationalOperator  RequirementInfo={} %GIDa_b5a4404b_9d12_499e_828e_45d226915324  Operator===  OutDataTypeStr=boolean  RndMeth=Nearest
  Relational Operator11 : RelationalOperator  RequirementInfo={} %GIDa_79c55e8f_6948_466a_9872_f547b9db4009  Operator===  OutDataTypeStr=boolean  RndMeth=Nearest
  Relational Operator12 : RelationalOperator  RequirementInfo={} %GIDa_17dec814_d961_4d3d_8cbf_fa9266c87c06  Operator===  OutDataTypeStr=boolean  RndMeth=Nearest
  Relational Operator13 : RelationalOperator  RequirementInfo={} %GIDa_77fa023d_9866_4d25_9e46_7da0f793e291  Operator===  OutDataTypeStr=boolean  RndMeth=Nearest
  Relational Operator14 : RelationalOperator  RequirementInfo={} %GIDa_d8f24c82_795e_4b5f_afa4_92e1340ebe13  Operator===  OutDataTypeStr=boolean  RndMeth=Nearest
  Relational Operator15 : RelationalOperator  RequirementInfo={} %GIDa_2e585a3d_30e2_4ac9_a524_28fc8b3f154b  Operator===  OutDataTypeStr=boolean  RndMeth=Nearest
  Relational Operator16 : RelationalOperator  RequirementInfo={} %GIDa_169954ed_64e0_40c9_accf_05b4d0a779dc  Operator===  OutDataTypeStr=boolean  RndMeth=Nearest
  Relational Operator2 : RelationalOperator  RequirementInfo={} %GIDa_74ed7b7b_e9e7_4b22_946c_9a0b388b4fd8  Operator===  OutDataTypeStr=boolean  RndMeth=Nearest
  Relational Operator3 : RelationalOperator  RequirementInfo={} %GIDa_d53e0909_38f3_4a1d_8d9d_2e2631c0bfd2  Operator===  OutDataTypeStr=boolean  RndMeth=Nearest
  Relational Operator4 : RelationalOperator  RequirementInfo={} %GIDa_b8bcb513_88af_4013_889f_2f7ba0e9afaa  Operator===  OutDataTypeStr=boolean  RndMeth=Nearest
  Relational Operator5 : RelationalOperator  RequirementInfo={} %GIDa_eae57311_6411_4570_9c95_6b21eeb45d86  Operator===  OutDataTypeStr=boolean  RndMeth=Nearest
  Relational Operator6 : RelationalOperator  RequirementInfo={} %GIDa_1a62504d_ac96_482e_ab94_0f36d2b37e2d  Operator===  OutDataTypeStr=boolean  RndMeth=Nearest
  Relational Operator7 : RelationalOperator  RequirementInfo={} %GIDa_c4efe30a_0353_437b_9881_24a86806ccce  Operator===  OutDataTypeStr=boolean  RndMeth=Nearest
  Relational Operator8 : RelationalOperator  RequirementInfo={} %GIDa_cbaf56e6_f0e0_4f5e_b0b1_1a89243fe511  Operator===  OutDataTypeStr=boolean  RndMeth=Nearest
  Relational Operator9 : RelationalOperator  RequirementInfo={} %GIDa_c7d52145_ac3e_4695_87e6_c47e08f80099  Operator===  OutDataTypeStr=boolean  RndMeth=Nearest
  Within Implies : sldvlib/Temporal Operators/Within Implies  RequirementInfo={} %GIDa_a850aec6_0f3a_409f_8ce3_0a4a0710d585  reset=off
      settings: SourceProductName=Simulink Design Verifier  SourceProductBaseCode=DV
  Within Implies1 : sldvlib/Temporal Operators/Within Implies  RequirementInfo={} %GIDa_a8c917f6_d6d4_49b6_a1ef_704c4073a93d  reset=off
      settings: SourceProductName=Simulink Design Verifier  SourceProductBaseCode=DV
  Within Implies2 : sldvlib/Temporal Operators/Within Implies  RequirementInfo={} %GIDa_5f44b74a_97d1_42a0_89ae_0fe79d0dd3f7  reset=off
      settings: SourceProductName=Simulink Design Verifier  SourceProductBaseCode=DV
  delayi1 : UnitDelay  RequirementInfo={} %GIDa_80ccc962_1e13_4ea5_8d86_e8a3cb862295  SampleTime=-1
  delayi2 : UnitDelay  RequirementInfo={} %GIDa_3b80eefc_c665_43bd_a5e3_3099e9de69d6  SampleTime=-1
  delayi3 : UnitDelay  RequirementInfo={} %GIDa_55d82d50_db91_437f_9a22_205827f00855  SampleTime=-1
  delayi4 : UnitDelay  RequirementInfo={} %GIDa_44646075_a9d3_4536_a4bb_2518e6127793  SampleTime=-1
  delayi5 : UnitDelay  RequirementInfo={} %GIDa_0913cb33_ff78_4736_9780_cf397ecef2d2  SampleTime=-1
  delayi6 : UnitDelay  RequirementInfo={} %GIDa_3e1d6896_ec7e_43d0_b858_377f9cbac27f  SampleTime=-1
  delayi7 : UnitDelay  RequirementInfo={} %GIDa_0eb5f02a_08dc_4a81_9a61_1e5499803556  SampleTime=-1
  gte1 : RelationalOperator  RequirementInfo={} %GIDa_58fdfaba_dbdd_4d96_820b_985e384d75dc  OutDataTypeStr=boolean  RndMeth=Nearest
  wires:
  delayi7/1 -> delayi4/1
  delayi6/1 -> delayi7/1
  Relational Operator16/1 -> delayi6/1
  delayi2/1 -> delayi3/1
  Relational Operator9/1 -> delayi2/1
  Constant12/1 -> Relational Operator10/2
  Relational Operator13/1 -> Logical Operator9/2
  Logical Operator8/1 -> Logical Operator10/1
  recoverable1/1 -> Relational Operator10/1
  Relational Operator14/1 -> Logical Operator8/2
  error1/1 -> Relational Operator14/1
  Implies2/1 -> Proof Objective5/1
  delayi5/1 -> Implies2/2
  Relational Operator12/1 -> Logical Operator9/1
  Detector1/1 -> Implies2/1
  Constant13/1 -> Relational Operator12/2
  Constant16/1 -> Relational Operator15/2
  Constant14/1 -> Relational Operator13/2
  Constant15/1 -> Relational Operator14/2
  Logical Operator9/1 -> Logical Operator8/1
  Logical Operator10/1 -> Detector1/1
  Relational Operator15/1 -> Logical Operator9/3
  Constant8/1 -> Relational Operator16/2
  delayi4/1 -> delayi5/1
  stateFlowModeLS4/1 -> Relational Operator16/1, Relational Operator12/1, Relational Operator13/1, Relational Operator15/1
  Relational Operator10/1 -> Logical Operator10/2
  Constant10/1 -> Relational Operator9/2
  task_error/1 -> Relational Operator9/1
  delayi3/1 -> Implies1/2
  Relational Operator11/1 -> Logical Operator7/2
  Logical Operator5/1 -> Logical Operator7/1
  Relational Operator7/1 -> Logical Operator5/2
  Constant7/1 -> Relational Operator7/2
  error/1 -> Relational Operator7/1
  Logical Operator6/1 -> Logical Operator5/1
  Relational Operator8/1 -> Logical Operator6/3
  Relational Operator5/1 -> Logical Operator6/2
  Relational Operator4/1 -> Logical Operator6/1
  Constant9/1 -> Relational Operator8/2
  Constant5/1 -> Relational Operator5/2
  Constant4/1 -> Relational Operator4/2
  stateFlowModeLS3/1 -> Relational Operator4/1, Relational Operator5/1, Relational Operator8/1
  Within Implies1/1 -> Proof Objective2/1
  Within Implies2/1 -> Proof Objective3/1
  Within Implies/1 -> Proof Objective1/1
  Detector3/1 -> Implies1/1
  Logical Operator7/1 -> Detector3/1
  recoverable/1 -> Relational Operator11/1
  Constant11/1 -> Relational Operator11/2
  Implies1/1 -> Proof Objective4/1
  load_counter/1 -> Within Implies2/2
  Constant6/1 -> Relational Operator6/1
  stateFlowModeLS2/1 -> Relational Operator2/1, Relational Operator6/2
  Constant3/1 -> Relational Operator2/2
  Relational Operator2/1 -> Delay6/1
  Relational Operator6/1 -> Logical Operator4/1
  Delay6/1 -> Logical Operator4/2
  Logical Operator4/1 -> Within Implies2/1
  Delay3/1 -> Logical Operator2/1
  Logical Operator3/1 -> Within Implies1/1
  Logical Operator1/1 -> Within Implies1/2
  Delay/1 -> Delay1/1
  Delay4/1 -> Delay2/1
  Relational Operator1/1 -> Logical Operator3/1
  Logical Operator2/1 -> Logical Operator1/3
  Delay2/1 -> Logical Operator1/2
  Constant1/1 -> Relational Operator1/2
  Delay5/1 -> Delay/1
  ctrl1/1 -> Delay5/1, Delay3/1, Delay4/1
  Delay1/1 -> Logical Operator/1
  stateFlowModeLS1/1 -> Relational Operator1/1
  increment/1 -> Logical Operator3/2
  Logical Operator/1 -> Logical Operator1/1
  inst_ptr/1 -> gte1/1, delayi1/1
  stateFlowModeLS/1 -> Relational Operator3/1
  delayi1/1 -> gte1/2
  Constant2/1 -> Relational Operator3/2
  gte1/1 -> Within Implies/2
  Relational Operator3/1 -> Within Implies/1

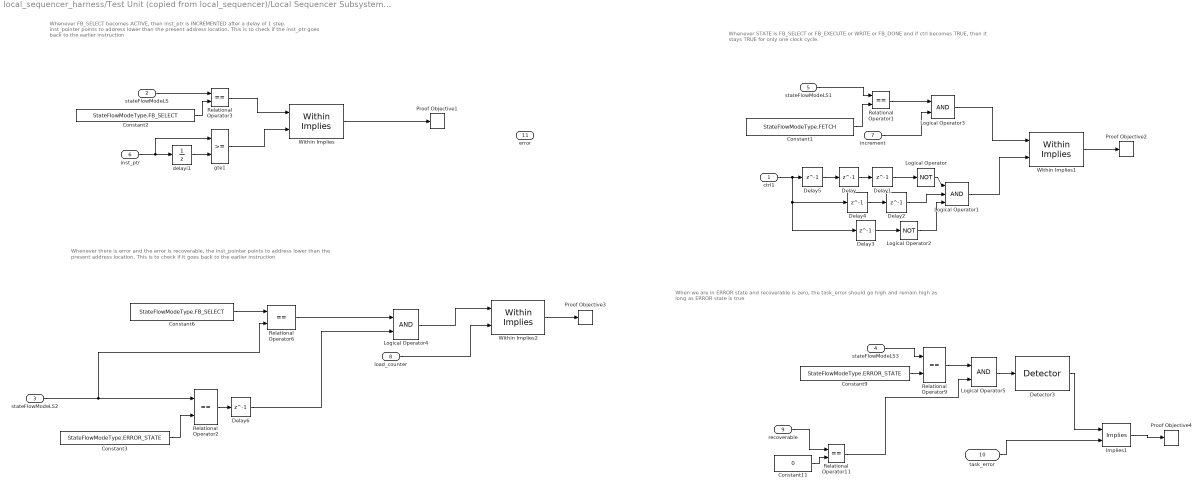
== system local_sequencer_harness/Test Unit (copied from local_sequencer)/Local Sequencer Subsystem/Verification Subsystem1 ==
  note: When we are in ERROR state and recoverable is zero, the task_error should go high and remain high as
      | long as ERROR state is true
  note: Whenever there is error and the error is recoverable, the inst_pointer points to address lower than the present address location. This is to check if it goes back to the earlier instruction
  note: Whenever STATE is FB_SELECT or FB_EXECUTE or WRITE or FB_DONE and if ctrl becomes TRUE, then it stays TRUE for only one clock cycle.
  note: Whenever FB_SELECT becomes ACTIVE, then inst_ptr is INCREMENTED after a delay of 1 step. inst_pointer points to address lower than the present address location. This is to check if the inst_ptr goes back to the earlier instruction
  ctrl1 : Inport  RequirementInfo={} %GIDa_da28b243_b868_43d7_ba2e_8c485d30471d
  stateFlowModeLS : Inport  RequirementInfo={} %GIDa_b658f277_eb35_4939_8a1c_f7bdb11b2e37  Port=2  OutDataTypeStr=Enum: StateFlowModeType
  stateFlowModeLS2 : Inport  RequirementInfo={} %GIDa_9494c7c7_948a_4f36_b45e_b32d219d933d  Port=3  OutDataTypeStr=Enum: StateFlowModeType
  stateFlowModeLS3 : Inport  RequirementInfo={} %GIDa_51971e87_c921_4f6d_98bc_24a46f192aa0  Port=4  OutDataTypeStr=Enum: StateFlowModeType
  stateFlowModeLS1 : Inport  RequirementInfo={} %GIDa_2205d377_0539_4f39_aa27_513b353afdfa  Port=5  OutDataTypeStr=Enum: StateFlowModeType
  inst_ptr : Inport  RequirementInfo={} %GIDa_e0198642_4de5_496c_8a1b_c80b9607f051  Port=6
  increment : Inport  RequirementInfo={} %GIDa_12f780a5_e4a5_4935_a5af_104c2ffef915  Port=7
  load_counter : Inport  RequirementInfo={} %GIDa_20c74391_262e_46b5_99fc_00060d204b47  Port=8
  recoverable : Inport  RequirementInfo={} %GIDa_767ccaa8_8cf2_4dec_8143_5926768f8cf1  Port=9
  task_error : Inport  RequirementInfo={} %GIDa_53cc32c6_315f_4191_931e_4b42866cfb7f  Port=10
  error : Inport  RequirementInfo={} %GIDa_d743bdee_6228_48aa_9015_424286047a7c  Port=11
  Constant1 : Constant  RequirementInfo={} %GIDa_08c62f4c_79dd_4aa1_8e1d_b7672b522beb  Value=StateFlowModeType.FETCH
  Constant11 : Constant  RequirementInfo={} %GIDa_e923a475_eeaa_4f5f_9d1f_bc779aa5a92f  Value=0
  Constant2 : Constant  RequirementInfo={} %GIDa_bdd20e68_8245_43a2_aee1_92fa65b992f0  Value=StateFlowModeType.FB_SELECT
  Constant3 : Constant  RequirementInfo={} %GIDa_32f9eb2f_8c35_4daf_a56f_79bbd1b75113  Value=StateFlowModeType.ERROR_STATE
  Constant6 : Constant  RequirementInfo={} %GIDa_22319c0a_c7bd_46dc_8f0e_1c43c9fbcbe1  Value=StateFlowModeType.FB_SELECT
  Constant9 : Constant  RequirementInfo={} %GIDa_a586b303_ff66_423a_928b_95e4785a77dc  Value=StateFlowModeType.ERROR_STATE
  Delay : Delay  RequirementInfo={} %GIDa_52c35e80_a692_43b0_ba0f_ba15d431e50d  DelayLength=1  InitialCondition=0
  Delay1 : Delay  RequirementInfo={} %GIDa_5edf2272_7f22_4436_8c63_712e735b9254  DelayLength=1  InitialCondition=0
  Delay2 : Delay  RequirementInfo={} %GIDa_ac1e625a_92e4_4437_b5dd_c8e8dfc2585e  DelayLength=1  InitialCondition=0
  Delay3 : Delay  RequirementInfo={} %GIDa_6882f156_e95a_4457_bff1_07e947ce6fe0  DelayLength=1  InitialCondition=0
  Delay4 : Delay  RequirementInfo={} %GIDa_dd209139_83cf_4834_9c80_2a839fc69b2d  DelayLength=1  InitialCondition=0
  Delay5 : Delay  RequirementInfo={} %GIDa_1b5d82ab_b22c_4a06_8248_ea3f7de96475  DelayLength=1  InitialCondition=0
  Delay6 : Delay  RequirementInfo={} %GIDa_66435e08_400f_4df3_8ae9_85f9d3d8a3b9  DelayLength=1  InitialCondition=0
  Detector3 : sldvlib/Temporal Operators/Detector  RequirementInfo={} %GIDa_9329c5e9_d204_4064_825a_267273615ea7  reset=off  typ=Synchronized  in_hold=1  delay=0  out_hold=5
      settings: SourceProductName=Simulink Design Verifier  SourceProductBaseCode=DV
  Implies1 : sldvlib/Verification Utilities/Implies  RequirementInfo={} %GIDa_9e3f4506_d330_49ca_92bc_f376778b2d46
      settings: SourceProductName=Simulink Design Verifier  SourceProductBaseCode=DV
  Logical Operator : Logic  RequirementInfo={} %GIDa_80c22c90_a824_4195_b7b4_018e449f4b98  Operator=NOT  AllPortsSameDT=off  OutDataTypeStr=boolean
  Logical Operator1 : Logic  RequirementInfo={} %GIDa_55f7f1b8_2cd4_4126_82d0_2a55cd03095a  Inputs=3  AllPortsSameDT=off  OutDataTypeStr=boolean
  Logical Operator2 : Logic  RequirementInfo={} %GIDa_b823976b_2aca_4db6_9281_208e03d05185  Operator=NOT  AllPortsSameDT=off  OutDataTypeStr=boolean
  Logical Operator3 : Logic  RequirementInfo={} %GIDa_43e37a52_d65d_4106_9b5e_fdf16ff6b511  AllPortsSameDT=off  OutDataTypeStr=boolean
  Logical Operator4 : Logic  RequirementInfo={} %GIDa_70c5bbdc_04cf_4f99_858c_f7f96b9a8a5e  AllPortsSameDT=off  OutDataTypeStr=boolean
  Logical Operator5 : Logic  RequirementInfo={} %GIDa_49fe060d_04d1_4504_a8c5_bbb9395ca26a  AllPortsSameDT=off  OutDataTypeStr=boolean
  Proof Objective1 : sldvlib/Objectives and Constraints/Proof Objective  RequirementInfo={} %GIDa_3e3bb8c9_c493_4881_9730_e999c58c5431  enabled=on  customAVTBlockType=Proof Objective  intervals=true  dispValues=on  outEnabled=off  enableStopSim=off
      settings: AttributesFormatString=%<intervals>  SourceProductName=Simulink Design Verifier  SourceProductBaseCode=DV
  Proof Objective2 : sldvlib/Objectives and Constraints/Proof Objective  RequirementInfo={} %GIDa_714c2f63_ef31_43d1_8117_59b66f4bc608  enabled=on  customAVTBlockType=Proof Objective  intervals=true  dispValues=on  outEnabled=off  enableStopSim=off
      settings: AttributesFormatString=%<intervals>  SourceProductName=Simulink Design Verifier  SourceProductBaseCode=DV
  Proof Objective3 : sldvlib/Objectives and Constraints/Proof Objective  RequirementInfo={} %GIDa_6b72de06_a2b0_461e_a7b5_bbf47dd6827b  enabled=on  customAVTBlockType=Proof Objective  intervals=true  dispValues=on  outEnabled=off  enableStopSim=off
      settings: AttributesFormatString=%<intervals>  SourceProductName=Simulink Design Verifier  SourceProductBaseCode=DV
  Proof Objective4 : sldvlib/Objectives and Constraints/Proof Objective  RequirementInfo={} %GIDa_57a76e19_0432_43dc_bf96_7defa76d949a  enabled=on  customAVTBlockType=Proof Objective  intervals=true  dispValues=on  outEnabled=off  enableStopSim=off
      settings: AttributesFormatString=%<intervals>  SourceProductName=Simulink Design Verifier  SourceProductBaseCode=DV
  Relational Operator1 : RelationalOperator  RequirementInfo={} %GIDa_3358586c_b492_4016_aee7_1cb0e8957062  Operator===  OutDataTypeStr=boolean  RndMeth=Nearest
  Relational Operator11 : RelationalOperator  RequirementInfo={} %GIDa_31529a48_961a_4cb2_8d8e_b059409aebbb  Operator===  OutDataTypeStr=boolean  RndMeth=Nearest
  Relational Operator2 : RelationalOperator  RequirementInfo={} %GIDa_33f66ad9_e82d_4cc8_a51b_8eb1737c8b5d  Operator===  OutDataTypeStr=boolean  RndMeth=Nearest
  Relational Operator3 : RelationalOperator  RequirementInfo={} %GIDa_21c71460_9e3f_4a8d_a43d_dd3ba93bd329  Operator===  OutDataTypeStr=boolean  RndMeth=Nearest
  Relational Operator6 : RelationalOperator  RequirementInfo={} %GIDa_5cd9b6ef_24f9_4bef_8ef6_ae7d7f845d71  Operator===  OutDataTypeStr=boolean  RndMeth=Nearest
  Relational Operator9 : RelationalOperator  RequirementInfo={} %GIDa_cb2bb49e_b979_4a3d_8a16_c85c8a383323  Operator===  OutDataTypeStr=boolean  RndMeth=Nearest
  Within Implies : sldvlib/Temporal Operators/Within Implies  RequirementInfo={} %GIDa_1bc41a05_dbb3_4197_9972_70c2618da667  reset=off
      settings: SourceProductName=Simulink Design Verifier  SourceProductBaseCode=DV
  Within Implies1 : sldvlib/Temporal Operators/Within Implies  RequirementInfo={} %GIDa_9d952d11_4398_44a0_9163_9b7e9caabb38  reset=off
      settings: SourceProductName=Simulink Design Verifier  SourceProductBaseCode=DV
  Within Implies2 : sldvlib/Temporal Operators/Within Implies  RequirementInfo={} %GIDa_1323bf0a_e7e0_4e51_8de3_7e2deddff203  reset=off
      settings: SourceProductName=Simulink Design Verifier  SourceProductBaseCode=DV
  delayi1 : UnitDelay  RequirementInfo={} %GIDa_cda4df61_1b45_49ba_9880_2a7ad5a5f824  SampleTime=-1
  gte1 : RelationalOperator  RequirementInfo={} %GIDa_f74728f1_59aa_4890_8c5e_e1edd53ed60f  OutDataTypeStr=boolean  RndMeth=Nearest
  wires:
  Within Implies1/1 -> Proof Objective2/1
  Within Implies2/1 -> Proof Objective3/1
  Within Implies/1 -> Proof Objective1/1
  Detector3/1 -> Implies1/1
  Logical Operator5/1 -> Detector3/1
  Relational Operator11/1 -> Logical Operator5/2
  recoverable/1 -> Relational Operator11/1
  Constant11/1 -> Relational Operator11/2
  Relational Operator9/1 -> Logical Operator5/1
  task_error/1 -> Implies1/2
  Implies1/1 -> Proof Objective4/1
  Constant9/1 -> Relational Operator9/2
  stateFlowModeLS3/1 -> Relational Operator9/1
  load_counter/1 -> Within Implies2/2
  Constant6/1 -> Relational Operator6/1
  stateFlowModeLS2/1 -> Relational Operator2/1, Relational Operator6/2
  Constant3/1 -> Relational Operator2/2
  Relational Operator2/1 -> Delay6/1
  Relational Operator6/1 -> Logical Operator4/1
  Delay6/1 -> Logical Operator4/2
  Logical Operator4/1 -> Within Implies2/1
  Delay3/1 -> Logical Operator2/1
  Logical Operator3/1 -> Within Implies1/1
  Logical Operator1/1 -> Within Implies1/2
  Delay/1 -> Delay1/1
  Delay4/1 -> Delay2/1
  Relational Operator1/1 -> Logical Operator3/1
  Logical Operator2/1 -> Logical Operator1/3
  Delay2/1 -> Logical Operator1/2
  Constant1/1 -> Relational Operator1/2
  Delay5/1 -> Delay/1
  ctrl1/1 -> Delay5/1, Delay3/1, Delay4/1
  Delay1/1 -> Logical Operator/1
  stateFlowModeLS1/1 -> Relational Operator1/1
  increment/1 -> Logical Operator3/2
  Logical Operator/1 -> Logical Operator1/1
  inst_ptr/1 -> gte1/1, delayi1/1
  stateFlowModeLS/1 -> Relational Operator3/1
  delayi1/1 -> gte1/2
  Constant2/1 -> Relational Operator3/2
  gte1/1 -> Within Implies/2
  Relational Operator3/1 -> Within Implies/1
